simulink model "I_controller_Different_KI_2Order"  (R2023b)
settings: Solver=VariableStepAuto  StartTime=0.0  StopTime=10.0  RelTol=1e-3
settings Model: Creator=ascom  LastModifiedBy=ascom

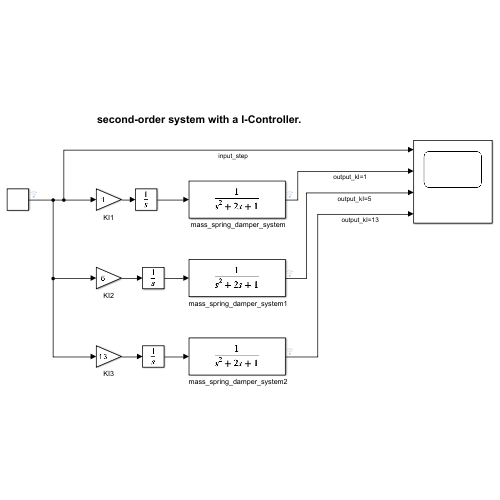
[thumbnail: Simulink's stored preview of the top-level diagram]
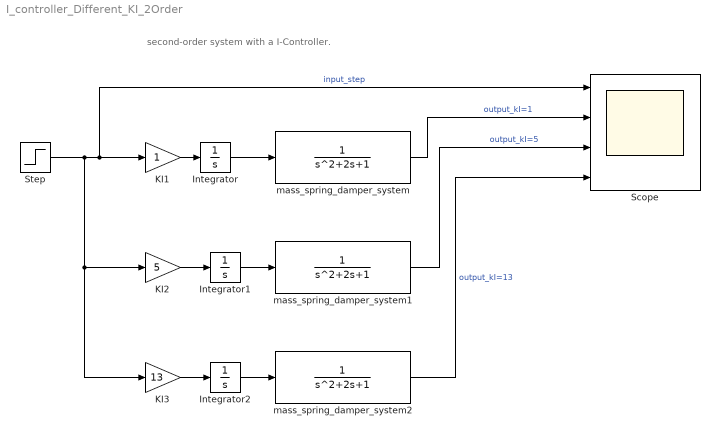
== system I_controller_Different_KI_2Order ==
  note: second-order system with a I-Controller.
  " mass_spring_damper_system" : TransferFcn
  " mass_spring_damper_system1" : TransferFcn
  " mass_spring_damper_system2" : TransferFcn
  Integrator : Integrator
  Integrator1 : Integrator
  Integrator2 : Integrator
  KI1 : Gain
  KI2 : Gain  Gain=5
  KI3 : Gain  Gain=13
  Scope : Scope  NumInputPorts=4
  Step : Step  SampleTime=0
  wires:
  " mass_spring_damper_system1"/1 -> Scope/3  "output_kI=5"
  KI2/1 -> Integrator1/1
  KI3/1 -> Integrator2/1
  " mass_spring_damper_system2"/1 -> Scope/4  "output_kI=13"
  Step/1 -> KI3/1, KI2/1, Scope/1, KI1/1  "input_step"
  " mass_spring_damper_system"/1 -> Scope/2  "output_kI=1"
  KI1/1 -> Integrator/1
  Integrator/1 -> " mass_spring_damper_system"/1
  Integrator1/1 -> " mass_spring_damper_system1"/1
  Integrator2/1 -> " mass_spring_damper_system2"/1
